simulink model "model"  (R2019a)
settings: Solver=VariableStepAuto  StartTime=0.0  StopTime=30  RelTol=1e-3
values from neighbouring files (symbols this model uses):
  B1 = (1/R1)+D1    (= 20.6)    [parameter.m]
  B2 = (1/R2)+D2    (= 16.9)    [parameter.m]
  D1 = 0.6    [parameter.m]
  D2 = 0.9    [parameter.m]
  fh = 100    [parameter.m]
  fl = 0.01    [parameter.m]
  M1 = 10    [parameter.m]
  M2 = 8    [parameter.m]
  R1 = 0.05    [parameter.m]
  R2 = 0.0625    [parameter.m]
  T12 = 1    [parameter.m]
  Tg1 = 0.2    [parameter.m]
  Tg2 = 0.3    [parameter.m]
  Tt1 = 0.5    [parameter.m]
  Tt2 = 0.6    [parameter.m]
  X_close = 0.4    [parameter.m]
  X_dash_close = 1.5    [parameter.m]
  X_dash_open = 0.4    [parameter.m]
  X_open = 1.2    [parameter.m]
undefined symbols (not defined in the file or in its folder): Kg
libraries: fod x2
settings Model: Creator=LENOVO  LastModifiedBy=LENOVO

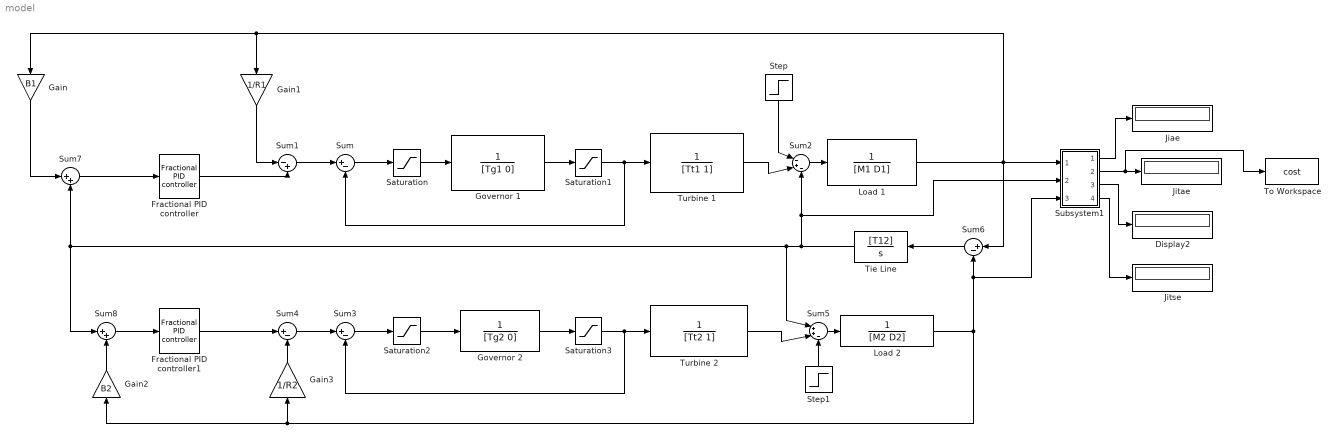
== system model ==
  Display2 : Display
  Fractional PID controller : fod/Fractional PID controller  Kp=Kg(1)  Ki=Kg(2)  lambda=Kg(4)  Kd=Kg(3)  mic=Kg(5)  freqRange=[2*pi*fl 2*pi*fh]  N=5
      settings: SourceProductName=FOMCON Toolbox
  Fractional PID controller1 : fod/Fractional PID controller  Kp=Kg(6)  Ki=Kg(7)  lambda=Kg(9)  Kd=Kg(8)  mic=Kg(10)  freqRange=[2*pi*fl 2*pi*fh]  N=5
      settings: SourceProductName=FOMCON Toolbox
  Gain : Gain  Gain=B1
  Gain1 : Gain  Gain=1/R1
  Gain2 : Gain  Gain=B2
  Gain3 : Gain  Gain=1/R2
  Governor 1 : TransferFcn  Denominator=[Tg1 0]
  Governor 2 : TransferFcn  Denominator=[Tg2 0]
  Jiae : Display
  Jitae : Display
  Jitse : Display
  Load 1 : TransferFcn  Denominator=[M1 D1]
  Load 2 : TransferFcn  Denominator=[M2 D2]
  Saturation : Saturate  UpperLimit=X_dash_open  LowerLimit=-1*X_dash_close
  Saturation1 : Saturate  UpperLimit=X_open  LowerLimit=-X_close
  Saturation2 : Saturate  UpperLimit=X_dash_open  LowerLimit=-1*X_dash_close
  Saturation3 : Saturate  UpperLimit=X_open  LowerLimit=-X_close
  Step : Step  Time=0  After=0.01  SampleTime=0
  Step1 : Step  Time=0  After=0.01  SampleTime=0
  Subsystem1 : Subsystem
  Sum{,3..4,6} (4 alike) : Sum  Inputs=|+-
  Sum1 : Sum  Inputs=|-+
  Sum2 : Sum  Inputs=|-+-
  Sum5 : Sum  Inputs=|++-
  Sum7 : Sum  Inputs=|++
  Sum8 : Sum  Inputs=|++
  Tie Line : TransferFcn  Numerator=[T12]  Denominator=[1 0]
  To Workspace : ToWorkspace  VariableName=cost  SampleTime=-1
  Turbine 1 : TransferFcn  Denominator=[Tt1 1]
  Turbine 2 : TransferFcn  Denominator=[Tt2 1]
  wires:
  Saturation/1 -> Governor 1/1
  Governor 1/1 -> Saturation1/1
  Saturation1/1 -> Sum/2, Turbine 1/1
  Sum/1 -> Saturation/1
  Sum1/1 -> Sum/1
  Sum2/1 -> Load 1/1
  Sum6/1 -> Tie Line/1
  Fractional PID controller/1 -> Sum1/2
  Sum7/1 -> Fractional PID controller/1
  Gain/1 -> Sum7/1
  Gain1/1 -> Sum1/1
  Sum8/1 -> Fractional PID controller1/1
  Sum5/1 -> Load 2/1
  Sum4/1 -> Sum3/1
  Sum3/1 -> Saturation2/1
  Saturation3/1 -> Sum3/2, Turbine 2/1
  Governor 2/1 -> Saturation3/1
  Saturation2/1 -> Governor 2/1
  Fractional PID controller1/1 -> Sum4/1
  Gain3/1 -> Sum4/2
  Gain2/1 -> Sum8/2
  Turbine 1/1 -> Sum2/2
  Turbine 2/1 -> Sum5/2
  Subsystem1/4(Jitse) -> Jitse/1
  Subsystem1/3(Jise) -> Display2/1
  Subsystem1/2(Jitae) -> To Workspace/1, Jitae/1
  Subsystem1/1(Jiae) -> Jiae/1
  Load 1/1 -> Sum6/1, Gain1/1, Gain/1, Subsystem1/1(Input)
  Tie Line/1 -> Sum8/1, Sum7/2, Sum5/1, Subsystem1/2(Input1), Sum2/3
  Load 2/1 -> Sum6/2, Subsystem1/3(Input2), Gain2/1, Gain3/1
  Step1/1 -> Sum5/3
  Step/1 -> Sum2/1

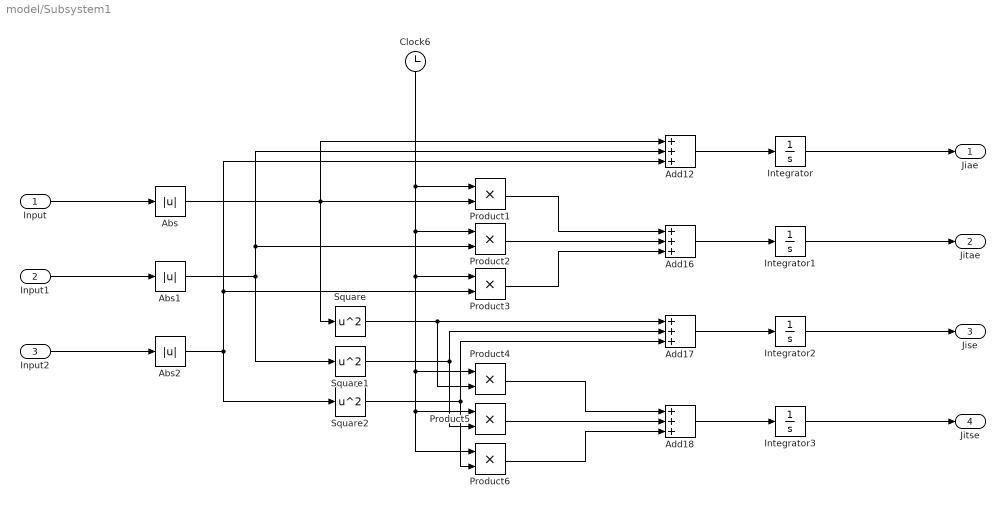
== system model/Subsystem1 ==
  Input : Inport
  Input1 : Inport  Port=2
  Input2 : Inport  Port=3
  Abs : Abs
  Abs1 : Abs
  Abs2 : Abs
  Add{12,16..18} (4 alike) : Sum  Inputs=+++
  Clock6 : Clock
  Integrator{,1..3} (4 alike) : Integrator
  Product{1..6} (6 alike) : Product
  Square : Math  Operator=square  SaturateOnIntegerOverflow=on
  Square1 : Math  Operator=square  SaturateOnIntegerOverflow=on
  Square2 : Math  Operator=square  SaturateOnIntegerOverflow=on
  Jiae : Outport
  Jitae : Outport  Port=2
  Jise : Outport  Port=3
  Jitse : Outport  Port=4
  wires:
  Input/1 -> Abs/1
  Product2/1 -> Add16/2
  Integrator1/1 -> Jitae/1
  Clock6/1 -> Product1/1, Product2/1, Product3/1, Product6/1, Product5/1, Product4/1
  Add16/1 -> Integrator1/1
  Integrator/1 -> Jiae/1
  Integrator2/1 -> Jise/1
  Integrator3/1 -> Jitse/1
  Product5/1 -> Add18/2
  Add18/1 -> Integrator3/1
  Add12/1 -> Integrator/1
  Input2/1 -> Abs2/1
  Square/1 -> Add17/1, Product4/2
  Product3/1 -> Add16/3
  Product6/1 -> Add18/3
  Input1/1 -> Abs1/1
  Square2/1 -> Add17/3, Product6/2
  Square1/1 -> Add17/2, Product5/2
  Product1/1 -> Add16/1
  Add17/1 -> Integrator2/1
  Product4/1 -> Add18/1
  Abs/1 -> Square/1, Add12/1, Product1/2
  Abs1/1 -> Add12/2, Product2/2, Square1/1
  Abs2/1 -> Square2/1, Add12/3, Product3/2
